simulink model "PID_Equation"  (R2020a)
settings: Solver=VariableStepAuto  StartTime=0.0  StopTime=10.0  RelTol=1e-3
undefined symbols (not defined in the file or in its folder): ki, kp, ts
settings Model: Creator=Ganesh  LastModifiedBy=Ganesh

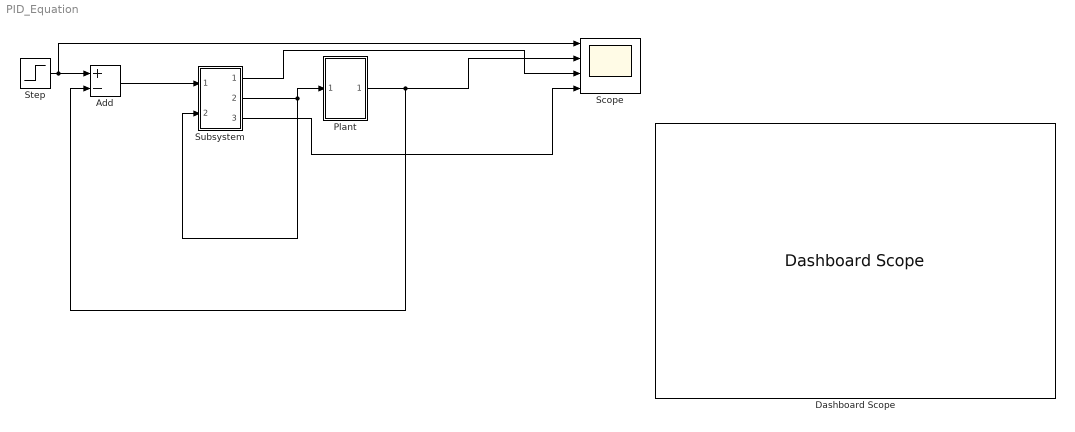
== system PID_Equation ==
  Add : Sum  Inputs=+-
  Dashboard Scope : DashboardScope
  Plant : Subsystem
  Scope : Scope  NumInputPorts=4
  Step : Step  Time=0  Before=-1  SampleTime=0
  Subsystem : Subsystem
  wires:
  Subsystem/1(Out1) -> Scope/3
  Subsystem/3(y[k]) -> Scope/4
  Subsystem/2(Out2) -> Subsystem/2(In2), Plant/1(In1)
  Plant/1(Out1) -> Add/2, Scope/2
  Step/1 -> Scope/1, Add/1
  Add/1 -> Subsystem/1(In1)

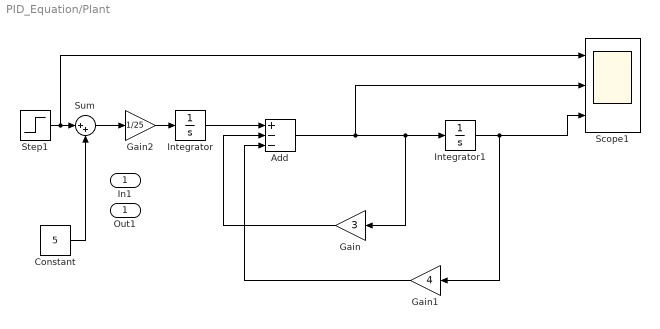
== system PID_Equation/Plant ==
  In1 : Inport
  Add : Sum  Inputs=+--
  Constant : Constant  Value=5
  Gain : Gain  Gain=3
  Gain1 : Gain  Gain=4
  Gain2 : Gain  Gain=1/25
  Integrator : Integrator
  Integrator1 : Integrator
  Scope1 : Scope  NumInputPorts=3
  Step1 : Step  SampleTime=0
  Sum : Sum  Inputs=|++
  Out1 : Outport
  wires:
  Gain/1 -> Add/2
  Integrator/1 -> Add/1
  Add/1 -> Scope1/2, Gain/1, Integrator1/1
  Integrator1/1 -> Scope1/3, Gain1/1
  Step1/1 -> Scope1/1, Sum/1
  Sum/1 -> Gain2/1
  Gain2/1 -> Integrator/1
  Constant/1 -> Sum/2
  Gain1/1 -> Add/3

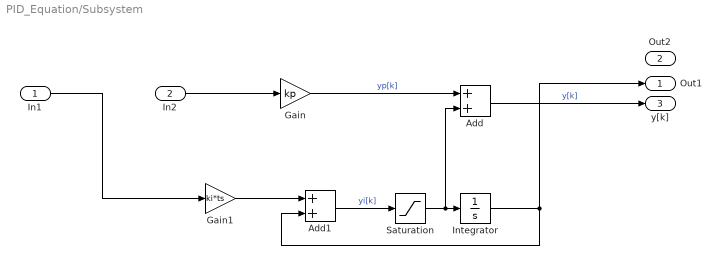
== system PID_Equation/Subsystem ==
  In1 : Inport
  In2 : Inport  Port=2
  Add : Sum
  Add1 : Sum
  Gain : Gain  Gain=kp
  Gain1 : Gain  Gain=ki*ts
  Integrator : Integrator
  Saturation : Saturate
  Out1 : Outport
  Out2 : Outport  Port=2
  y[k] : Outport  Port=3
  wires:
  Add1/1 -> Saturation/1  "yi[k]"
  Gain1/1 -> Add1/1
  In2/1 -> Gain/1
  Integrator/1 -> Out1/1, Add1/2
  Saturation/1 -> Add/2, Integrator/1
  In1/1 -> Gain1/1
  Add/1 -> y[k]/1  "y[k]"
  Gain/1 -> Add/1  "yp[k]"
